simulink model "FlexibleJointRobots_Catalogue"  (R2020b)
settings: Solver=VariableStepAuto  StartTime=0.0  StopTime=10  RelTol=1e-4
undefined symbols (not defined in the file): init
settings Model: Creator=mdxavier  LastModifiedBy=mdxavier

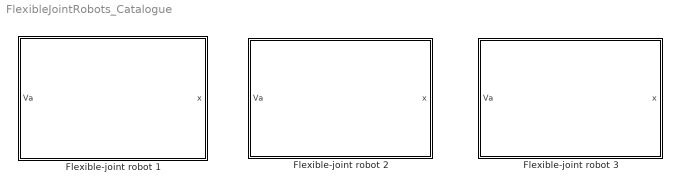
== system FlexibleJointRobots_Catalogue ==
  Flexible-joint robot 1 : Subsystem
      mask Display: image('$imagefile'); % Use "Edit Image" on toolstrip to change.
  Flexible-joint robot 2 : Subsystem
      mask Display: image('$imagefile'); % Use "Edit Image" on toolstrip to change.
  Flexible-joint robot 3 : Subsystem
      mask Display: image('$imagefile'); % Use "Edit Image" on toolstrip to change.

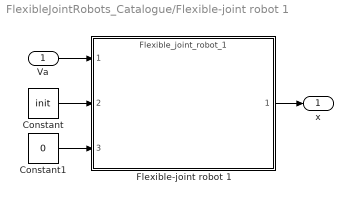
== system FlexibleJointRobots_Catalogue/Flexible-joint robot 1 ==
  Va : Inport
  Constant : Constant  Value=init
  Constant1 : Constant  Value=0
  Flexible-joint robot 1 : ModelReference  ModelNameDialog=Flexible_joint_robot_1  ModelReferenceVersion=1.65  CopyOfModelProtected=on
  x : Outport
  wires:
  Constant/1 -> Flexible-joint robot 1/2
  Constant1/1 -> Flexible-joint robot 1/3
  Flexible-joint robot 1/1 -> x/1
  Va/1 -> Flexible-joint robot 1/1

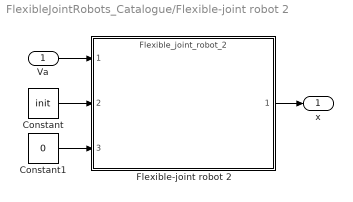
== system FlexibleJointRobots_Catalogue/Flexible-joint robot 2 ==
  Va : Inport
  Constant : Constant  Value=init
  Constant1 : Constant  Value=0
  Flexible-joint robot 2 : ModelReference  ModelNameDialog=Flexible_joint_robot_2  ModelReferenceVersion=1.65  CopyOfModelProtected=on
  x : Outport
  wires:
  Va/1 -> Flexible-joint robot 2/1
  Constant1/1 -> Flexible-joint robot 2/3
  Constant/1 -> Flexible-joint robot 2/2
  Flexible-joint robot 2/1 -> x/1

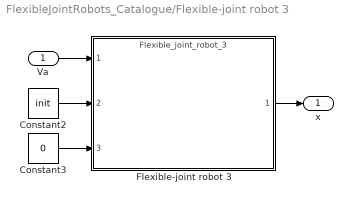
== system FlexibleJointRobots_Catalogue/Flexible-joint robot 3 ==
  Va : Inport
  Constant2 : Constant  Value=init
  Constant3 : Constant  Value=0
  Flexible-joint robot 3 : ModelReference  ModelNameDialog=Flexible_joint_robot_3  ModelReferenceVersion=1.65  CopyOfModelProtected=on
  x : Outport
  wires:
  Flexible-joint robot 3/1 -> x/1
  Constant2/1 -> Flexible-joint robot 3/2
  Constant3/1 -> Flexible-joint robot 3/3
  Va/1 -> Flexible-joint robot 3/1
